simulink model "secondoModello"  (R2024a)
settings: Solver=FixedStepAuto  StartTime=0.0  StopTime=inf  RelTol=1e-3
libraries: dspsrcs4 x3, dspsnks4 x1, dspfdesign x1
settings Model: Creator=Alessandro  LastModifiedBy=Alessandro

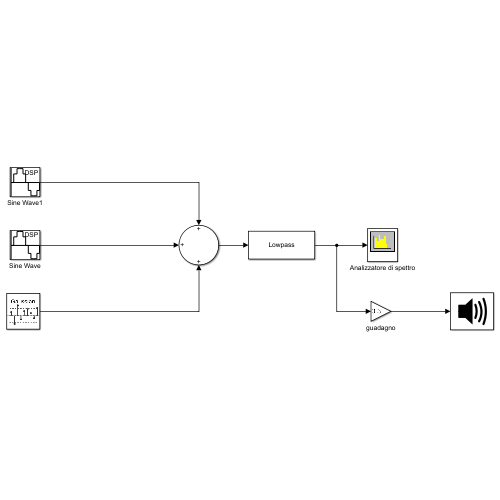
[thumbnail: Simulink's stored preview of the top-level diagram]
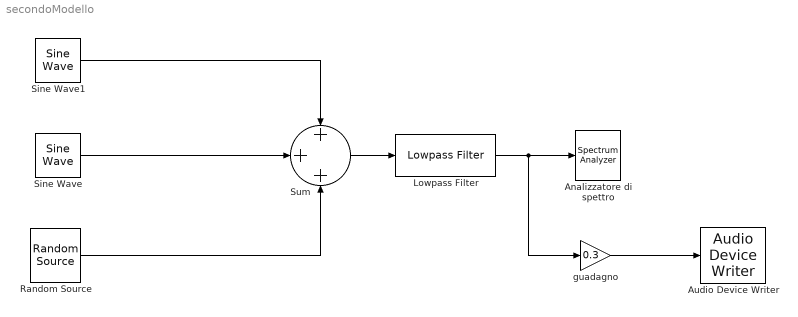
== system secondoModello ==
  Analizzatore di spettro : SpectrumAnalyzer  WindowPosition=[207.000000,89.000000,800.000000,500.000000,]  ScopeFrameLocation=window  SampleRateSource=Property  SampleRate=44.1e3  PlotAsTwoSidedSpectrum=off  FrequencyScale=Log  FrequencySpan=Start and stop frequencies  StartFrequency=20  StopFrequency=20e3  YLimits=[-68.56730733,41.24730984]  SelectedToolstripTab=spectrumAnalyzerToolstrip.channelMeasurementsTab
  Audio Device Writer : dspsnks4/Audio Device Writer  Driver=DirectSound  Device=Altoparlanti (TOPPING USB DAC)  InheritSampleRate=on  SampleRate=44100  BitDepth=24-bit integer  BufferSize=4096  NumBuffers=10  DefaultOutputChannelMapping=on  OutputChannelMapping=1:2  OutputNumUnderrunSamples=off  DriverIdx=1  DeviceWarnFlag=''
  Lowpass Filter : dspfdesign/Lowpass Filter  FilterType=FIR  DesignForMinimumOrder=on  FilterOrder=50  PassbandFrequency=600  StopbandFrequency=900  PassbandRipple=1  StopbandAttenuation=60  SampleRateMode=Specify on dialog  SampleRate=48000  SimulateUsing=Interpreted execution  roundingMode=Floor  coeffsDataTypeStr=fixdt(1,16)
  Random Source : dspsrcs4/Random Source  SrcType=Gaussian  MinVal=0  MaxVal=1  MeanVal=0  VarVal=1  RepMode=Specify seed  rawSeed=1  IsInherit=off  SampTime=1  SampFrame=1  OutComplex=Real  DataType=double  SimulateUsing=Interpreted execution
  Sine Wave : dspsrcs4/Sine Wave  Amplitude=1  Frequency=500  Phase=1000  SampleMode=Discrete  OutComplex=Real  CompMethod=Trigonometric fcn  TableSize=Speed  SampleTime=1/48000  SamplesPerFrame=1  ResetState=Restart at time zero  OutputFrames=off  dataType=double  wordLen=16  udDataType=sfix(16)  fracBitsMode=Best precision  numFracBits=15  OutDataTypeStr=double  LastOutDataTypeStr=double
  Sine Wave1 : dspsrcs4/Sine Wave  Amplitude=1  Frequency=500  Phase=1000  SampleMode=Discrete  OutComplex=Real  CompMethod=Trigonometric fcn  TableSize=Speed  SampleTime=1/48000  SamplesPerFrame=1  ResetState=Restart at time zero  OutputFrames=off  dataType=double  wordLen=16  udDataType=sfix(16)  fracBitsMode=Best precision  numFracBits=15  OutDataTypeStr=double  LastOutDataTypeStr=double
  Sum : Sum  Inputs=+++
  guadagno : Gain  Gain=0.3
  wires:
  Lowpass Filter/1 -> Analizzatore di spettro/1, guadagno/1
  Sine Wave1/1 -> Sum/1
  Sine Wave/1 -> Sum/2
  Random Source/1 -> Sum/3
  guadagno/1 -> Audio Device Writer/1
  Sum/1 -> Lowpass Filter/1
